simulink model "untitled"  (R2024a)
settings: Solver=VariableStepAuto  StartTime=0.0  StopTime=10.0  RelTol=1e-3
settings Model: Creator=dhyeyfindoriya  LastModifiedBy=dhyeyfindoriya

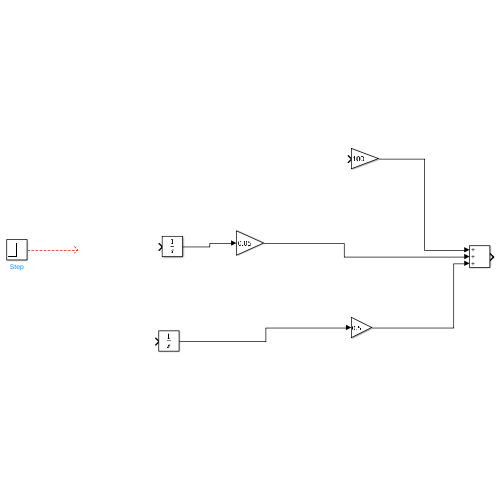
[thumbnail: Simulink's stored preview of the top-level diagram]
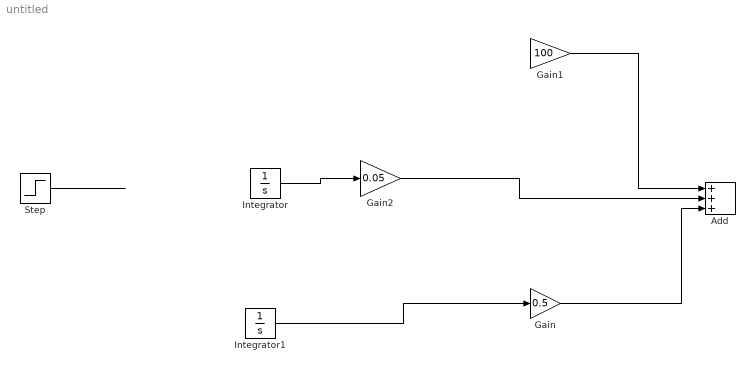
== system untitled ==
  Add : Sum  Inputs=+++
  Gain : Gain  Gain=0.5
  Gain1 : Gain  Gain=100
  Gain2 : Gain  Gain=0.05
  Integrator : Integrator
  Integrator1 : Integrator
  Step : Step  SampleTime=0
  wires:
  Step/1 -> ?
  Gain/1 -> Add/3
  Gain1/1 -> Add/1
  Gain2/1 -> Add/2
  Integrator1/1 -> Gain/1
  Integrator/1 -> Gain2/1
